simulink model "VehicleBicycleModel"  (R2018b)
settings: Solver=VariableStepAuto  StartTime=0.0  StopTime=10.0  RelTol=1e-3
libraries: autolibshared x5, vehdynlibtirecommon x2, autolibutils x2, sharedtransform x1
(part 1 of 4)
settings Model: Creator=ivory  LastModifiedBy=ivory

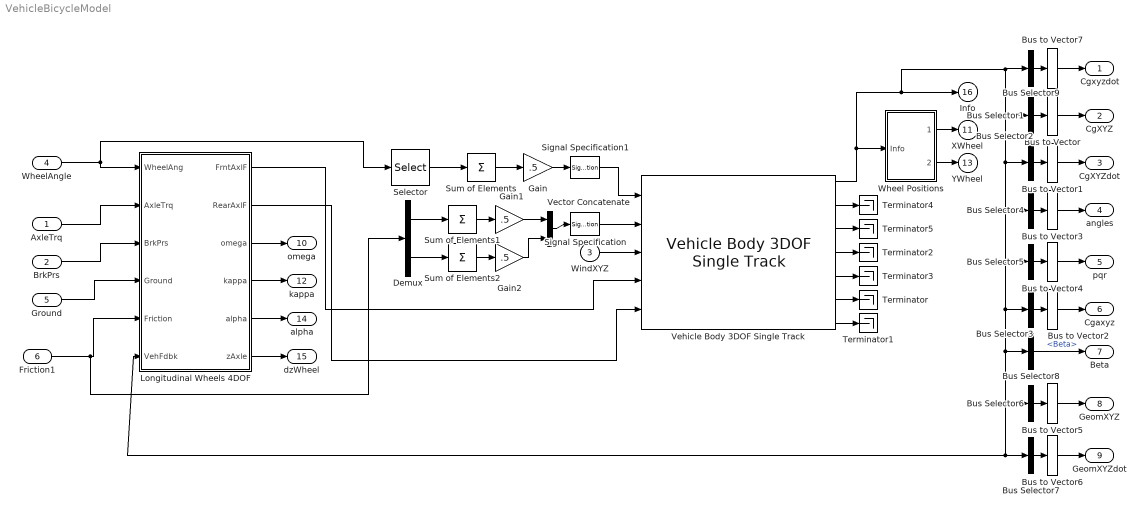
== system VehicleBicycleModel ==
  AxleTrq : Inport  Unit=N*m  PortDimensions=4
  BrkPrs : Inport  Port=2  Unit=Pa  PortDimensions=4
  WindXYZ : Inport  Port=3
  WheelAngle : Inport  Port=4  Unit=rad  PortDimensions=4
  Ground : Inport  Port=5  Unit=m  PortDimensions=4
  Friction1 : Inport  Port=6  Unit=1  PortDimensions=4
  Bus Selector1 : BusSelector  OutputSignals=InertFrm.Cg.Disp.X,InertFrm.Cg.Disp.Y,InertFrm.Cg.Disp.Z  OutputAsBus=on
  Bus Selector2 : BusSelector  OutputSignals=InertFrm.Cg.Vel.Xdot,InertFrm.Cg.Vel.Ydot,InertFrm.Cg.Vel.Zdot  OutputAsBus=on
  Bus Selector3 : BusSelector  OutputSignals=BdyFrm.Cg.Acc.ax,BdyFrm.Cg.Acc.ay,BdyFrm.Cg.Acc.az  OutputAsBus=on
  Bus Selector4 : BusSelector  OutputSignals=InertFrm.Cg.Ang.phi,InertFrm.Cg.Ang.theta,InertFrm.Cg.Ang.psi  OutputAsBus=on
  Bus Selector5 : BusSelector  OutputSignals=BdyFrm.Cg.AngVel.p,BdyFrm.Cg.AngVel.q,BdyFrm.Cg.AngVel.r  OutputAsBus=on
  Bus Selector6 : BusSelector  OutputSignals=InertFrm.Geom.Disp.X,InertFrm.Geom.Disp.Y,InertFrm.Geom.Disp.Z  OutputAsBus=on
  Bus Selector7 : BusSelector  OutputSignals=InertFrm.Geom.Vel.Xdot,InertFrm.Geom.Vel.Ydot,InertFrm.Geom.Vel.Zdot  OutputAsBus=on
  Bus Selector8 : BusSelector  OutputSignals=BdyFrm.Geom.Ang.Beta
  Bus Selector9 : BusSelector  OutputSignals=BdyFrm.Cg.Vel.xdot,BdyFrm.Cg.Vel.ydot,BdyFrm.Cg.Vel.zdot  OutputAsBus=on
  Bus to Vector{,1..7} (8 alike) : BusToVector
  Demux : Demux  Outputs=[2,2]
  Gain : Gain  Gain=.5
  Gain1 : Gain  Gain=.5
  Gain2 : Gain  Gain=.5
  Longitudinal Wheels 4DOF : Subsystem  VariantControl=1  mask{wheelMode=Single track (bicycle)}
      mask prompts: wheelMode "Wheel mode:"
      settings: AttributesFormatString=%<wheelMode>
      mask TypeOptions wheelMode: Single track (bicycle) | Dual track
      mask Callback wheelMode:
      | switch get_param(gcb,'wheelMode')
      |     case 'Single track (bicycle)'
      |         set_param([bdroot '/Longitudinal Wheels 4DOF/Velocity and Vertical Load'],'OverrideUsingVariant','0')
      |         set_param([bdroot '/Longitudinal Wheels 4DOF/Axle Forces'],'OverrideUsingVariant','0')
      |     case 'Dual track'
      |         set_param([bdroot '/Longitudinal Wheels 4DOF/Velocity and Vertical Load'],'OverrideUsingVariant','1')
      |         set_param([bdroot '/Longitudinal Wheels 4DOF/Axle Forces'],'OverrideUsingVariant','1')
      |     otherwise
      |         set_param([bdroot '/Longitudinal Wheels 4DOF/Velocity and Vertical Load'],'OverrideUsingVariant','0')
      |         set_param([bdroot '/Longitudinal Wheels 4DOF/Axle Forces'],'OverrideUsingVariant','0')
      | end
  Selector : Selector  InputPortWidth=4  IndexOptions=Index vector (dialog)  Indices=[1 2]  OutputSizes=1
  Signal Specification : SignalSpecification  Unit=1
  Signal Specification1 : SignalSpecification  Unit=rad
  Sum of Elements : Sum  Inputs=+
  Sum of Elements1 : Sum  Inputs=+
  Sum of Elements2 : Sum  Inputs=+
  Terminator{,1..5} (6 alike) : Terminator
  Vector Concatenate : Concatenate
  Vehicle Body 3DOF Single Track : autolibshared/Vehicle Body 3DOF Single Track  trackMode=Single (bicycle)  inputMode=External longitudinal forces  frontSteerMode=on  rearSteerMode=off  windMode=on  muMode=on  extFMode=off  extMMode=off  aMode=2  NF=2  NR=2  m=1181  a=1.515  b=1.5040  h=0.1340  X_o=0  xdot_o=0  CalphaMode=off  sigmaMode=on  d=0  w=1.922.*[1 1]  Cy_f=15000  Cy_r=35000  sigma_f=.1  sigma_r=.1  alpha_f_brk=[-.1 .1]  Cy_f_data=[-9e3 9e3]  alpha_r_brk=[-.1 .1]  Cy_r_data=[-9e3 9e3]  Y_o=3.1250  ydot_o=0  Izz=2066  psi_o=0  r_o=0  Af=2.11  Cd=.3  Cl=.1  Cpm=.1  beta_w=[0:0.01:0.3]  Cs=[0:0.03:0.9]  Cym=[0:0.01:0.3]  Pabs=101325  Tair=273  g=9.81  mu=1  xdot_tol=1  Fznom=5000  Fxtire_sat=7e3*1e3  Fytire_sat=2e3*1e3  longOff=0  latOff=0  vertOff=.0112
      settings: SourceProductName=Powertrain Blockset  SourceProductBaseCode=PW
  Wheel Positions : Subsystem
  Cgxyzdot : Outport
  CgXYZ : Outport  Port=2
  CgXYZdot : Outport  Port=3
  angles : Outport  Port=4
  pqr : Outport  Port=5
  Cgaxyz : Outport  Port=6
  Beta : Outport  Port=7
  GeomXYZ : Outport  Port=8
  GeomXYZdot : Outport  Port=9  Unit=m/s
  omega : Outport  Port=10  PortDimensions=4
  XWheel : Outport  Port=11  Unit=m
  kappa : Outport  Port=12  PortDimensions=4
  " YWheel" : Outport  Port=13  Unit=m
  alpha : Outport  Port=14  PortDimensions=4
  dzWheel : Outport  Port=15
  " Info" : Outport  Port=16
  wires:
  Vehicle Body 3DOF Single Track/6 -> Terminator/1
  Longitudinal Wheels 4DOF/2(RearAxlF) -> Vehicle Body 3DOF Single Track/5
  Signal Specification1/1 -> Vehicle Body 3DOF Single Track/1
  Signal Specification/1 -> Vehicle Body 3DOF Single Track/2
  Sum of Elements/1 -> Gain/1
  Vehicle Body 3DOF Single Track/3 -> Terminator5/1
  Gain/1 -> Signal Specification1/1
  Demux/1 -> Sum of Elements1/1
  Wheel Positions/1(XWheel) -> XWheel/1
  Sum of Elements1/1 -> Gain1/1
  WindXYZ/1 -> Vehicle Body 3DOF Single Track/3
  Vehicle Body 3DOF Single Track/5 -> Terminator3/1
  WheelAngle/1 -> Selector/1, Longitudinal Wheels 4DOF/1(WheelAng)
  Vehicle Body 3DOF Single Track/4 -> Terminator2/1
  Vehicle Body 3DOF Single Track/7 -> Terminator1/1
  Vehicle Body 3DOF Single Track/2 -> Terminator4/1
  Vector Concatenate/1 -> Signal Specification/1
  Longitudinal Wheels 4DOF/1(FrntAxlF) -> Vehicle Body 3DOF Single Track/4
  Wheel Positions/2(YWheel) -> " YWheel"/1
  Gain2/1 -> Vector Concatenate/2
  Selector/1 -> Sum of Elements/1
  Demux/2 -> Sum of Elements2/1
  Friction1/1 -> Longitudinal Wheels 4DOF/5(Friction), Demux/1
  Gain1/1 -> Vector Concatenate/1
  Sum of Elements2/1 -> Gain2/1
  Bus to Vector2/1 -> Cgaxyz/1
  Vehicle Body 3DOF Single Track/1 -> Bus Selector8/1, Bus Selector6/1, Longitudinal Wheels 4DOF/6(VehFdbk), Bus Selector7/1, Bus Selector3/1, Bus Selector5/1, Bus Selector4/1, Bus Selector2/1, Bus Selector1/1, Bus Selector9/1, " Info"/1, Wheel Positions/1(Info)
  Bus Selector3/1 -> Bus to Vector2/1
  Bus to Vector/1 -> CgXYZ/1
  Bus Selector2/1 -> Bus to Vector1/1
  Bus Selector6/1 -> Bus to Vector5/1
  Bus to Vector4/1 -> pqr/1
  Bus to Vector5/1 -> GeomXYZ/1
  Bus Selector5/1 -> Bus to Vector4/1
  Bus Selector7/1 -> Bus to Vector6/1
  Bus Selector4/1 -> Bus to Vector3/1
  Bus to Vector1/1 -> CgXYZdot/1
  Bus Selector1/1 -> Bus to Vector/1
  Bus to Vector7/1 -> Cgxyzdot/1
  Bus to Vector6/1 -> GeomXYZdot/1
  Bus Selector8/1 -> Beta/1  "<Beta>"
  Bus Selector9/1 -> Bus to Vector7/1
  Bus to Vector3/1 -> angles/1
  Longitudinal Wheels 4DOF/3(omega) -> omega/1
  Longitudinal Wheels 4DOF/4(kappa) -> kappa/1
  Longitudinal Wheels 4DOF/5(alpha) -> alpha/1
  Longitudinal Wheels 4DOF/6(zAxle) -> dzWheel/1
  AxleTrq/1 -> Longitudinal Wheels 4DOF/2(AxleTrq)
  BrkPrs/1 -> Longitudinal Wheels 4DOF/3(BrkPrs)
  Ground/1 -> Longitudinal Wheels 4DOF/4(Ground)

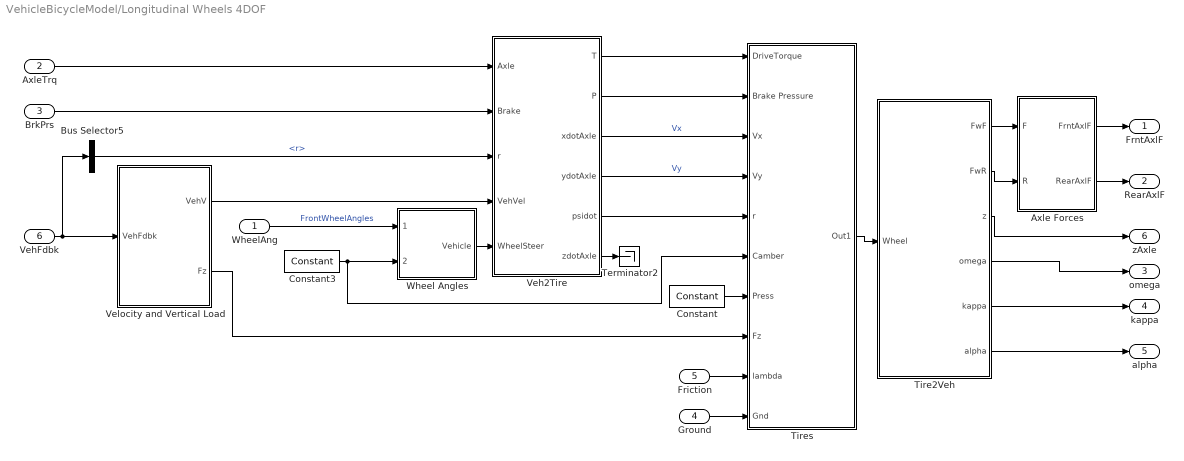
== system VehicleBicycleModel/Longitudinal Wheels 4DOF ==
  WheelAng : Inport
  AxleTrq : Inport  Port=2
  BrkPrs : Inport  Port=3
  Ground : Inport  Port=4  PortDimensions=4
  Friction : Inport  Port=5  PortDimensions=4
  VehFdbk : Inport  Port=6
  Axle Forces : Subsystem  VariantControlMode=Label  Variant=on  LabelModeActiveChoice=0
  Bus Selector5 : BusSelector  OutputSignals=BdyFrm.Cg.AngVel.r
  Constant : vehdynlibtirecommon/Constant  const=220000  numWheels=4
  Constant3 : vehdynlibtirecommon/Constant  const=0  numWheels=4
  Terminator2 : Terminator
  Tire2Veh : Subsystem
  Tires : Subsystem
  Veh2Tire : Subsystem
  Velocity and Vertical Load : Subsystem  VariantControlMode=Label  Variant=on  LabelModeActiveChoice=0
  Wheel Angles : Subsystem
  FrntAxlF : Outport  Unit=N
  RearAxlF : Outport  Port=2  Unit=N
  omega : Outport  Port=3
  kappa : Outport  Port=4
  alpha : Outport  Port=5
  zAxle : Outport  Port=6
  wires:
  Wheel Angles/1(Vehicle) -> Veh2Tire/5(WheelSteer)
  Tires/1(Out1) -> Tire2Veh/1(Wheel)
  Friction/1 -> Tires/9(lambda)
  Constant/1 -> Tires/7(Press)
  Constant3/1 -> Wheel Angles/2(Camber), Tires/6(Camber)
  Veh2Tire/3(xdotAxle) -> Tires/3(Vx)  "Vx"
  Ground/1 -> Tires/10(Gnd)
  VehFdbk/1 -> Bus Selector5/1, Velocity and Vertical Load/1(VehFdbk)
  AxleTrq/1 -> Veh2Tire/1(Axle)
  Veh2Tire/1(T) -> Tires/1(DriveTorque)
  Veh2Tire/2(P) -> Tires/2(Brake Pressure)
  BrkPrs/1 -> Veh2Tire/2(Brake)
  Bus Selector5/1 -> Veh2Tire/3(r)  "<r>"
  Veh2Tire/6(zdotAxle) -> Terminator2/1
  WheelAng/1 -> Wheel Angles/1(WheelAng)  "FrontWheelAngles"
  Veh2Tire/4(ydotAxle) -> Tires/4(Vy)  "Vy"
  Veh2Tire/5(psidot) -> Tires/5(r)
  Velocity and Vertical Load/2(Fz) -> Tires/8(Fz)
  Velocity and Vertical Load/1(VehV) -> Veh2Tire/4(VehVel)
  Axle Forces/1(FrntAxlF) -> FrntAxlF/1
  Axle Forces/2(RearAxlF) -> RearAxlF/1
  Tire2Veh/1(FwF) -> Axle Forces/1(F)
  Tire2Veh/2(FwR) -> Axle Forces/2(R)
  Tire2Veh/3(z) -> zAxle/1
  Tire2Veh/4(omega) -> omega/1
  Tire2Veh/5(kappa) -> kappa/1
  Tire2Veh/6(alpha) -> alpha/1

== system VehicleBicycleModel/Wheel Positions ==
  Info : Inport
  Bus Selector : BusSelector  OutputSignals=InertFrm.FrntAxl.Disp.Y,InertFrm.RearAxl.Disp.Y
  Bus Selector1 : BusSelector  OutputSignals=InertFrm.FrntAxl.Disp.X,InertFrm.RearAxl.Disp.X
  Ground : Ground
  Ground1 : Ground
  Vector Concatenate1 : Concatenate  NumInputs=4
  Vector Concatenate2 : Concatenate  NumInputs=4
  XWheel : Outport  Unit=m
  YWheel : Outport  Port=2  Unit=m
  wires:
  Ground/1 -> Vector Concatenate1/4, Vector Concatenate1/2
  Vector Concatenate1/1 -> YWheel/1
  Bus Selector/2 -> Vector Concatenate1/3  "<Y>"
  Bus Selector/1 -> Vector Concatenate1/1  "<Y>"
  Ground1/1 -> Vector Concatenate2/4, Vector Concatenate2/2
  Info/1 -> Bus Selector/1, Bus Selector1/1
  Vector Concatenate2/1 -> XWheel/1
  Bus Selector1/2 -> Vector Concatenate2/3  "<X>"
  Bus Selector1/1 -> Vector Concatenate2/1  "<X>"

== system VehicleBicycleModel/Longitudinal Wheels 4DOF/Axle Forces ==
  note: 1) Add Subsystem or Model blocks as valid variant choices.
      | 2) You cannot connect blocks at this level. At simulation, connectivity is automatically
      | determined, based on the active variant and port name matching.
  F : Inport
  R : Inport  Port=2
  Bicycle : Subsystem  VariantControl=0
  Dual : Subsystem  VariantControl=1
  FrntAxlF : Outport  Unit=N
  RearAxlF : Outport  Port=2  Unit=N

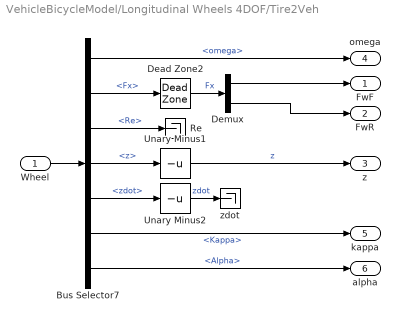
== system VehicleBicycleModel/Longitudinal Wheels 4DOF/Tire2Veh ==
  Wheel : Inport
  Bus Selector7 : BusSelector  OutputSignals=omega,Fx,Re,z,zdot,Kappa,Alpha
  Dead Zone2 : DeadZone  LowerValue=-5  UpperValue=5  ZeroCross=off  SaturateOnIntegerOverflow=on
  Demux : Demux  Outputs=[2,2]
  Re : Terminator
  Unary Minus1 : UnaryMinus
  Unary Minus2 : UnaryMinus
  zdot : Terminator
  FwF : Outport
  FwR : Outport  Port=2
  z : Outport  Port=3
  omega : Outport  Port=4
  kappa : Outport  Port=5
  alpha : Outport  Port=6
  wires:
  Bus Selector7/2 -> Dead Zone2/1  "<Fx>"
  Dead Zone2/1 -> Demux/1  "Fx"
  Demux/1 -> FwF/1
  Wheel/1 -> Bus Selector7/1
  Bus Selector7/1 -> omega/1  "<omega>"
  Bus Selector7/5 -> Unary Minus2/1  "<zdot>"
  Bus Selector7/4 -> Unary Minus1/1  "<z>"
  Unary Minus1/1 -> z/1  "z"
  Demux/2 -> FwR/1
  Bus Selector7/6 -> kappa/1  "<Kappa>"
  Unary Minus2/1 -> zdot/1  "zdot"
  Bus Selector7/3 -> Re/1  "<Re>"
  Bus Selector7/7 -> alpha/1  "<Alpha>"
